simulink model "torqueWalking"  (Simulink 8.9)
settings: Solver=FixedStepDiscrete  StartTime=0.0  StopTime=Config.t_end  FixedStep=Config.t_step  RelTol=1e-3  EnableMultiTasking=on
InitFcn:
  | cd(fileparts(which(bdroot)));
  | initTorqueWalkingMPC;
undefined symbols (not defined in the file or in its folder): biasVectorConstraint_feet, Config, ConstraintMatrix_feet, DiscIntNeverNeededParam, Gains, ROBOT_DOF, Sat
libraries: WBToolboxLibrary x101
(part 1 of 3)
settings Model: SuppressorTable=22 serialization::archive 11 0 6 0 0 0 11 0  Creator=gnava  LastModifiedBy=mcharbonneau
settings DataIOCC: LimitDataPoints=off  SaveFormat=Dataset  SignalLoggingSaveFormat=Dataset
settings OptimizationCC: LifeSpan=auto
settings DebuggingCC: UnderspecifiedInitializationDetection=Simplified  MergeDetectMultiDrivingBlocksExec=error  FcnCallInpInsideContextMsg=error  StateNameClashWarn=none  SFUnexpectedBacktrackingDiag=error  SFNoUnconditionalDefaultTransitionDiag=error
settings HardwareCC: ProdBitPerPointer=64  ProdBitPerSizeT=64  ProdBitPerPtrDiffT=64  ProdLargestAtomicFloat=Float  ProdIntDivRoundTo=Zero  ProdEndianess=LittleEndian  ProdWordSize=64  ProdHWDeviceType=Intel->x86-64 (Windows64)
settings ModelReferenceCC: PropagateSignalLabelsOutOfModel=on
settings GRTTargetCC: TargetLangStandard=C99 (ISO)  GeneratePreprocessorConditionals=Use local settings  CombineOutputUpdateFcns=on  GRTInterface=off
settings ConfigComp: CovSFcnEnable=off

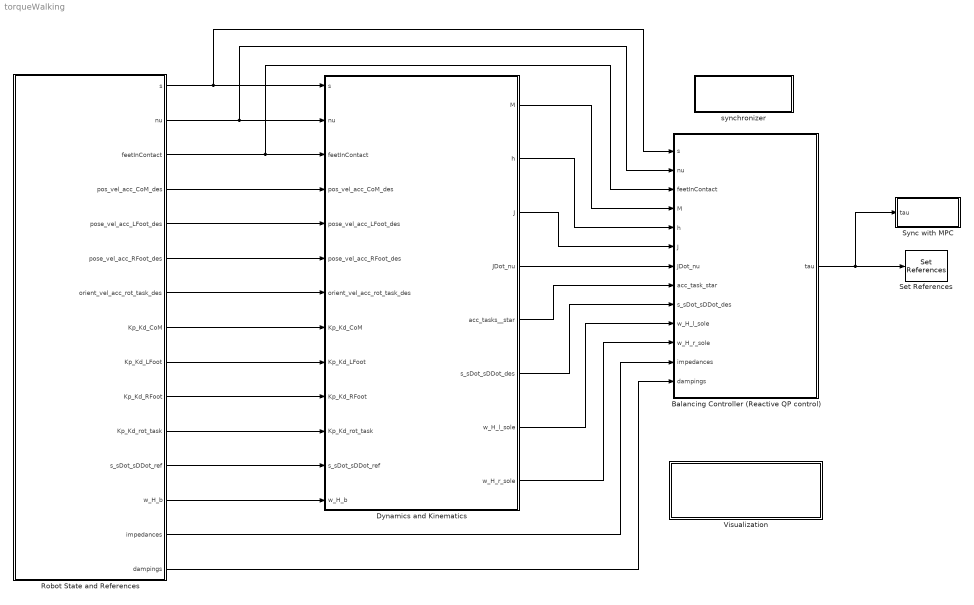
== system torqueWalking ==
  Balancing Controller (Reactive QP control) : Subsystem
  Dynamics and Kinematics : Subsystem
  Robot State and References : Subsystem
  Set References : WBToolboxLibrary/wholeBodyActuators/Set References  controlType=Torque  fullOrSubControl=Full  controlledJoints=''  robotName=WBT_robotName  localName=WBT_modelName  wbiFile=WBT_wbiFilename  wbiList=WBT_wbiList
      settings: SourceProductName=Whole Body Toolbox
  Sync with MPC : Subsystem
      mask Display: disp('Sync with MPC')
  Visualization : Subsystem
      mask Display: disp('VISUALIZE AND DUMP DATA')
  synchronizer : Subsystem
      mask Display: disp('SYNCHRONIZER')
  wires:
  Robot State and References/2(nu) -> Dynamics and Kinematics/2(nu), Balancing Controller (Reactive QP control)/2(nu)
  Robot State and References/3(feetInContact) -> Balancing Controller (Reactive QP control)/3(feetInContact), Dynamics and Kinematics/3(feetInContact)
  Robot State and References/4(pos_vel_acc_CoM_des) -> Dynamics and Kinematics/4(pos_vel_acc_CoM_des)
  Robot State and References/5(pose_vel_acc_LFoot_des) -> Dynamics and Kinematics/5(pose_vel_acc_LFoot_des)
  Robot State and References/6(pose_vel_acc_RFoot_des) -> Dynamics and Kinematics/6(pose_vel_acc_RFoot_des)
  Robot State and References/7(orient_vel_acc_rot_task_des) -> Dynamics and Kinematics/7(orient_vel_acc_rot_task_des)
  Robot State and References/8(Kp_Kd_CoM) -> Dynamics and Kinematics/8(Kp_Kd_CoM)
  Robot State and References/9(Kp_Kd_LFoot) -> Dynamics and Kinematics/9(Kp_Kd_LFoot)
  Robot State and References/10(Kp_Kd_RFoot) -> Dynamics and Kinematics/10(Kp_Kd_RFoot)
  Robot State and References/11(Kp_Kd_rot_task) -> Dynamics and Kinematics/11(Kp_Kd_rot_task)
  Robot State and References/12(s_sDot_sDDot_ref) -> Dynamics and Kinematics/12(s_sDot_sDDot_ref)
  Robot State and References/13(w_H_b) -> Dynamics and Kinematics/13(w_H_b)
  Dynamics and Kinematics/4(JDot_nu) -> Balancing Controller (Reactive QP control)/7(JDot_nu)
  Robot State and References/1(s) -> Dynamics and Kinematics/1(s), Balancing Controller (Reactive QP control)/1(s)
  Dynamics and Kinematics/1(M) -> Balancing Controller (Reactive QP control)/4(M)
  Dynamics and Kinematics/2(h) -> Balancing Controller (Reactive QP control)/5(h)
  Dynamics and Kinematics/3(J) -> Balancing Controller (Reactive QP control)/6(J)
  Balancing Controller (Reactive QP control)/1(tau) -> Sync with MPC/1(tau), Set References/1
  Dynamics and Kinematics/5(acc_tasks__star) -> Balancing Controller (Reactive QP control)/8(acc_task_star)
  Dynamics and Kinematics/6(s_sDot_sDDot_des) -> Balancing Controller (Reactive QP control)/9(s_sDot_sDDot_des)
  Dynamics and Kinematics/7(w_H_l_sole) -> Balancing Controller (Reactive QP control)/10(w_H_l_sole)
  Dynamics and Kinematics/8(w_H_r_sole) -> Balancing Controller (Reactive QP control)/11(w_H_r_sole)
  Robot State and References/14(impedances) -> Balancing Controller (Reactive QP control)/12(impedances)
  Robot State and References/15(dampings) -> Balancing Controller (Reactive QP control)/13(dampings)

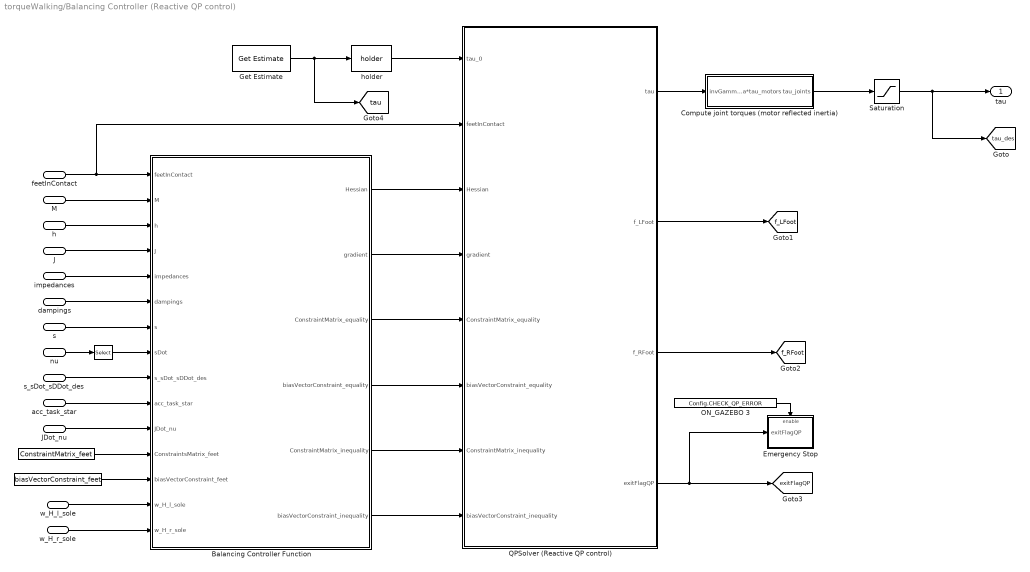
== system torqueWalking/Balancing Controller (Reactive QP control) ==
  s : Inport
  nu : Inport  Port=2
  feetInContact : Inport  Port=3
  M : Inport  Port=4
  h : Inport  Port=5
  J : Inport  Port=6
  JDot_nu : Inport  Port=7
  acc_task_star : Inport  Port=8
  s_sDot_sDDot_des : Inport  Port=9
  w_H_l_sole : Inport  Port=10
  w_H_r_sole : Inport  Port=11
  impedances : Inport  Port=12
  dampings : Inport  Port=13
  "   " : Constant  Value=ConstraintMatrix_feet
  "      " : Constant  Value=biasVectorConstraint_feet
  "             " : Selector  InputPortWidth=ROBOT_DOF+6  IndexOptions=Index vector (dialog)  Indices=[7:ROBOT_DOF+6]  OutputSizes=1
  Balancing Controller Function : MATLAB Function  TreatAsAtomicUnit=on
  Compute joint torques (motor reflected inertia) : Subsystem
  Emergency Stop : Subsystem
  Get Estimate : WBToolboxLibrary/wholeBodyStates/Get Estimate  estimateType=Joints Torque  robotName=WBT_robotName  localName=WBT_modelName  wbiFile=WBT_wbiFilename  wbiList=WBT_wbiList
      settings: SourceProductName=Whole Body Toolbox
  ON_GAZEBO 3 : Constant  Value=Config.CHECK_QP_ERROR
  QPSolver (Reactive QP control) : Subsystem
  Saturation : Saturate  UpperLimit=Sat.tau_max  LowerLimit=-Sat.tau_max
  "holder " : WBToolboxLibrary/Utilities/holder 
      settings: SourceProductName=Whole Body Toolbox
  tau : Outport
  tag scope: exitFlagQP=global, f_LFoot=global, f_RFoot=global, tau=global, tau_des=global
  wires:
  QPSolver (Reactive QP control)/1(tau) -> Compute joint torques (motor reflected inertia)/1(invGamma*tau_motors)
  "holder "/1 -> QPSolver (Reactive QP control)/1(tau_0)
  Balancing Controller Function/3(ConstraintMatrix_equality) -> QPSolver (Reactive QP control)/5(ConstraintMatrix_equality)
  Balancing Controller Function/6(biasVectorConstraint_inequality) -> QPSolver (Reactive QP control)/8(biasVectorConstraint_inequality)
  Balancing Controller Function/2(gradient) -> QPSolver (Reactive QP control)/4(gradient)
  Balancing Controller Function/4(biasVectorConstraint_equality) -> QPSolver (Reactive QP control)/6(biasVectorConstraint_equality)
  Balancing Controller Function/5(ConstraintMatrix_inequality) -> QPSolver (Reactive QP control)/7(ConstraintMatrix_inequality)
  w_H_r_sole/1 -> Balancing Controller Function/15(w_H_r_sole)
  w_H_l_sole/1 -> Balancing Controller Function/14(w_H_l_sole)
  "      "/1 -> Balancing Controller Function/13(biasVectorConstraint_feet)
  "   "/1 -> Balancing Controller Function/12(ConstraintsMatrix_feet)
  JDot_nu/1 -> Balancing Controller Function/11(JDot_nu)
  acc_task_star/1 -> Balancing Controller Function/10(acc_task_star)
  s_sDot_sDDot_des/1 -> Balancing Controller Function/9(s_sDot_sDDot_des)
  nu/1 -> "             "/1
  s/1 -> Balancing Controller Function/7(s)
  dampings/1 -> Balancing Controller Function/6(dampings)
  impedances/1 -> Balancing Controller Function/5(impedances)
  J/1 -> Balancing Controller Function/4(J)
  h/1 -> Balancing Controller Function/3(h)
  M/1 -> Balancing Controller Function/2(M)
  Get Estimate/1 -> [tau], "holder "/1
  "             "/1 -> Balancing Controller Function/8(sDot)
  Saturation/1 -> tau/1, [tau_des]
  Balancing Controller Function/1(Hessian) -> QPSolver (Reactive QP control)/3(Hessian)
  feetInContact/1 -> Balancing Controller Function/1(feetInContact), QPSolver (Reactive QP control)/2(feetInContact)
  QPSolver (Reactive QP control)/2(f_LFoot) -> [f_LFoot]
  QPSolver (Reactive QP control)/3(f_RFoot) -> [f_RFoot]
  QPSolver (Reactive QP control)/4(exitFlagQP) -> Emergency Stop/1(exitFlagQP), [exitFlagQP]
  ON_GAZEBO 3/1 -> Emergency Stop/Enable
  Compute joint torques (motor reflected inertia)/1(tau_joints) -> Saturation/1

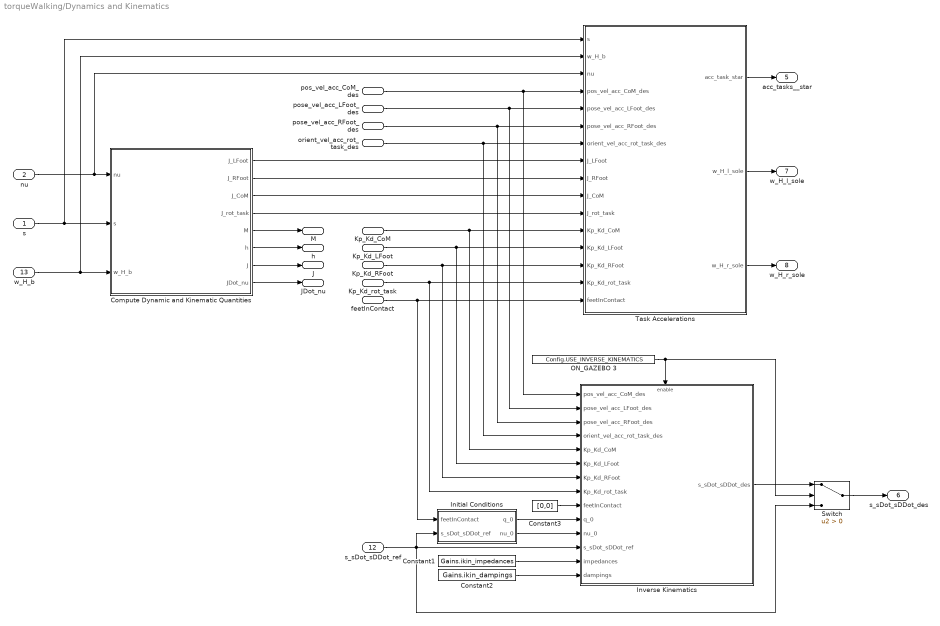
== system torqueWalking/Dynamics and Kinematics ==
  s : Inport
  nu : Inport  Port=2
  feetInContact : Inport  Port=3
  pos_vel_acc_CoM_des : Inport  Port=4
  pose_vel_acc_LFoot_des : Inport  Port=5
  pose_vel_acc_RFoot_des : Inport  Port=6
  orient_vel_acc_rot_task_des : Inport  Port=7
  Kp_Kd_CoM : Inport  Port=8
  Kp_Kd_LFoot : Inport  Port=9
  Kp_Kd_RFoot : Inport  Port=10
  Kp_Kd_rot_task : Inport  Port=11
  s_sDot_sDDot_ref : Inport  Port=12
  w_H_b : Inport  Port=13
  Compute Dynamic and Kinematic Quantities : Subsystem
  Constant1 : Constant  Value=Gains.ikin_impedances
  Constant2 : Constant  Value=Gains.ikin_dampings
  Constant3 : Constant  Value=[0,0]
  Initial Conditions : Subsystem
  Inverse Kinematics : Subsystem
  ON_GAZEBO 3 : Constant  Value=Config.USE_INVERSE_KINEMATICS
  Switch : Switch  Criteria=u2 > Threshold
  Task Accelerations : Subsystem
  M : Outport
  h : Outport  Port=2
  J : Outport  Port=3
  JDot_nu : Outport  Port=4
  acc_tasks__star : Outport  Port=5
  s_sDot_sDDot_des : Outport  Port=6
  w_H_l_sole : Outport  Port=7
  w_H_r_sole : Outport  Port=8
  wires:
  pos_vel_acc_CoM_des/1 -> Task Accelerations/4(pos_vel_acc_CoM_des), Inverse Kinematics/1(pos_vel_acc_CoM_des)
  pose_vel_acc_LFoot_des/1 -> Task Accelerations/5(pose_vel_acc_LFoot_des), Inverse Kinematics/2(pose_vel_acc_LFoot_des)
  pose_vel_acc_RFoot_des/1 -> Task Accelerations/6(pose_vel_acc_RFoot_des), Inverse Kinematics/3(pose_vel_acc_RFoot_des)
  orient_vel_acc_rot_task_des/1 -> Task Accelerations/7(orient_vel_acc_rot_task_des), Inverse Kinematics/4(orient_vel_acc_rot_task_des)
  Kp_Kd_CoM/1 -> Task Accelerations/12(Kp_Kd_CoM), Inverse Kinematics/5(Kp_Kd_CoM)
  Kp_Kd_LFoot/1 -> Task Accelerations/13(Kp_Kd_LFoot), Inverse Kinematics/6(Kp_Kd_LFoot)
  Kp_Kd_RFoot/1 -> Task Accelerations/14(Kp_Kd_RFoot), Inverse Kinematics/7(Kp_Kd_RFoot)
  Kp_Kd_rot_task/1 -> Task Accelerations/15(Kp_Kd_rot_task), Inverse Kinematics/8(Kp_Kd_rot_task)
  Task Accelerations/1(acc_task_star) -> acc_tasks__star/1
  ON_GAZEBO 3/1 -> Switch/2, Inverse Kinematics/Enable
  Inverse Kinematics/1(s_sDot_sDDot_des) -> Switch/1
  nu/1 -> Compute Dynamic and Kinematic Quantities/1(nu), Task Accelerations/3(nu)
  s/1 -> Task Accelerations/1(s), Compute Dynamic and Kinematic Quantities/2(s)
  w_H_b/1 -> Compute Dynamic and Kinematic Quantities/3(w_H_b), Task Accelerations/2(w_H_b)
  Compute Dynamic and Kinematic Quantities/6(h) -> h/1
  Compute Dynamic and Kinematic Quantities/1(J_LFoot) -> Task Accelerations/8(J_LFoot)
  Compute Dynamic and Kinematic Quantities/2(J_RFoot) -> Task Accelerations/9(J_RFoot)
  Compute Dynamic and Kinematic Quantities/3(J_CoM) -> Task Accelerations/10(J_CoM)
  Compute Dynamic and Kinematic Quantities/5(M) -> M/1
  Compute Dynamic and Kinematic Quantities/4(J_rot_task) -> Task Accelerations/11(J_rot_task)
  Compute Dynamic and Kinematic Quantities/7(J) -> J/1
  Compute Dynamic and Kinematic Quantities/8(JDot_nu) -> JDot_nu/1
  s_sDot_sDDot_ref/1 -> Switch/3, Inverse Kinematics/12(s_sDot_sDDot_ref), Initial Conditions/2(s_sDot_sDDot_ref)
  Initial Conditions/1(q_0) -> Inverse Kinematics/10(q_0)
  Initial Conditions/2(nu_0) -> Inverse Kinematics/11(nu_0)
  Constant1/1 -> Inverse Kinematics/13(impedances)
  Constant2/1 -> Inverse Kinematics/14(dampings)
  Switch/1 -> s_sDot_sDDot_des/1
  Constant3/1 -> Inverse Kinematics/9(feetInContact)
  feetInContact/1 -> Initial Conditions/1(feetInContact), Task Accelerations/16(feetInContact)
  Task Accelerations/2(w_H_l_sole) -> w_H_l_sole/1
  Task Accelerations/3(w_H_r_sole) -> w_H_r_sole/1

== system torqueWalking/Robot State and References ==
  Gain Scheduling : Subsystem
  "Smooth References " : Subsystem
  State Machines : Subsystem
  s : Outport
  nu : Outport  Port=2
  feetInContact : Outport  Port=3
  pos_vel_acc_CoM_des : Outport  Port=4
  pose_vel_acc_LFoot_des : Outport  Port=5
  pose_vel_acc_RFoot_des : Outport  Port=6
  orient_vel_acc_rot_task_des : Outport  Port=7
  Kp_Kd_CoM : Outport  Port=8
  Kp_Kd_LFoot : Outport  Port=9
  Kp_Kd_RFoot : Outport  Port=10
  Kp_Kd_rot_task : Outport  Port=11
  s_sDot_sDDot_ref : Outport  Port=12
  w_H_b : Outport  Port=13
  impedances : Outport  Port=14
  dampings : Outport  Port=15
  wires:
  Gain Scheduling/1(Kp_Kd_CoM) -> Kp_Kd_CoM/1
  Gain Scheduling/2(Kp_Kd_LFoot) -> Kp_Kd_LFoot/1
  Gain Scheduling/3(Kp_Kd_RFoot) -> Kp_Kd_RFoot/1
  Gain Scheduling/4(Kp_Kd_rot_task) -> Kp_Kd_rot_task/1
  Gain Scheduling/5(impedances) -> impedances/1
  Gain Scheduling/6(dampings) -> dampings/1
  State Machines/5(state) -> Gain Scheduling/1(state), "Smooth References "/1(state)
  State Machines/4(feetInContact) -> feetInContact/1
  State Machines/3(nu) -> nu/1
  State Machines/2(w_H_b) -> w_H_b/1
  State Machines/6(references_CoM) -> "Smooth References "/2(references_CoM)
  State Machines/7(references_LFoot) -> "Smooth References "/3(references_LFoot)
  State Machines/8(references_RFoot) -> "Smooth References "/4(references_RFoot)
  State Machines/9(references_rot_task) -> "Smooth References "/5(references_rot_task)
  State Machines/10(references_s) -> "Smooth References "/6(references_s)
  "Smooth References "/1(pos_vel_acc_CoM_des) -> pos_vel_acc_CoM_des/1
  "Smooth References "/2(pose_vel_acc_LFoot_des) -> pose_vel_acc_LFoot_des/1
  "Smooth References "/3(pose_vel_acc_RFoot_des) -> pose_vel_acc_RFoot_des/1
  "Smooth References "/4(orient_vel_acc_rot_task_des) -> orient_vel_acc_rot_task_des/1
  "Smooth References "/5(s_sDot_sDDot_ref) -> s_sDot_sDDot_ref/1
  State Machines/1(s) -> s/1

== system torqueWalking/Sync with MPC ==
  tau : Inport
  Clock : Clock
  Gain : Gain  Gain=0
  Mux : Mux  Inputs=2
  Selector : Selector  InputPortWidth=ROBOT_DOF  IndexOptions=Index vector (dialog)  Indices=[1]  OutputSizes=1
  Yarp Write : WBToolboxLibrary/Utilities/Yarp Write  portName=PORTS.ACK  autoconnect=on  errorOnConnection=off
      settings: SourceProductName=Whole Body Toolbox
  wires:
  Clock/1 -> Mux/2
  tau/1 -> Selector/1
  Mux/1 -> Yarp Write/1
  Selector/1 -> Gain/1
  Gain/1 -> Mux/1

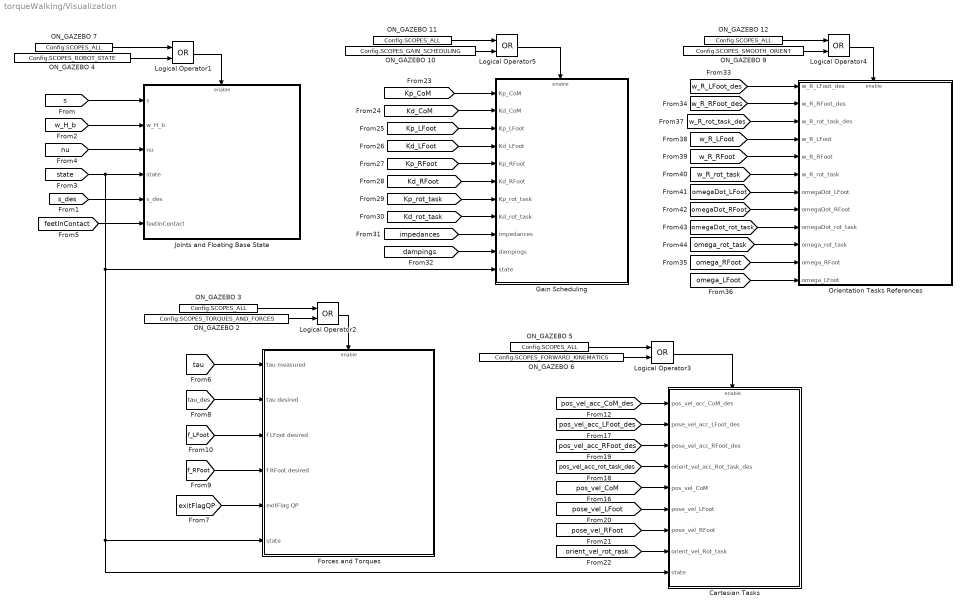
== system torqueWalking/Visualization ==
  Cartesian Tasks : Subsystem
  Forces and Torques : Subsystem
  Gain Scheduling : Subsystem
  Joints and Floating Base State : Subsystem
  Logical Operator{1..5} (5 alike) : Logic  Operator=OR  AllPortsSameDT=off  OutDataTypeStr=boolean
  ON_GAZEBO 10 : Constant  Value=Config.SCOPES_GAIN_SCHEDULING
  ON_GAZEBO {3,5,7,11..12} (5 alike) : Constant  Value=Config.SCOPES_ALL
  ON_GAZEBO 2 : Constant  Value=Config.SCOPES_TORQUES_AND_FORCES
  ON_GAZEBO 4 : Constant  Value=Config.SCOPES_ROBOT_STATE
  ON_GAZEBO 6 : Constant  Value=Config.SCOPES_FORWARD_KINEMATICS
  ON_GAZEBO 9 : Constant  Value=Config.SCOPES_SMOOTH_ORIENT
  Orientation Tasks References : Subsystem
  wires:
  [s] -> Joints and Floating Base State/1(s)
  [w_H_b] -> Joints and Floating Base State/2(w_H_b)
  [s_des] -> Joints and Floating Base State/5(s_des)
  [nu] -> Joints and Floating Base State/3(nu)
  [state] -> Cartesian Tasks/9(state), Forces and Torques/6(state), Gain Scheduling/11(state), Joints and Floating Base State/4(state)
  [tau] -> Forces and Torques/1(tau measured)
  [tau_des] -> Forces and Torques/2(tau desired)
  [f_LFoot] -> Forces and Torques/3(f LFoot desired)
  [f_RFoot] -> Forces and Torques/4(f RFoot desired)
  [exitFlagQP] -> Forces and Torques/5(exitFlag QP)
  ON_GAZEBO 4/1 -> Logical Operator1/2
  ON_GAZEBO 7/1 -> Logical Operator1/1
  Logical Operator1/1 -> Joints and Floating Base State/Enable
  [feetInContact] -> Joints and Floating Base State/6(feetInContact)
  Logical Operator2/1 -> Forces and Torques/Enable
  ON_GAZEBO 3/1 -> Logical Operator2/1
  ON_GAZEBO 2/1 -> Logical Operator2/2
  ON_GAZEBO 6/1 -> Logical Operator3/2
  Logical Operator3/1 -> Cartesian Tasks/Enable
  ON_GAZEBO 5/1 -> Logical Operator3/1
  [pos_vel_acc_CoM_des] -> Cartesian Tasks/1(pos_vel_acc_CoM_des)
  [pos_vel_acc_LFoot_des] -> Cartesian Tasks/2(pose_vel_acc_LFoot_des)
  [pos_vel_acc_RFoot_des] -> Cartesian Tasks/3(pose_vel_acc_RFoot_des)
  [pos_vel_acc_rot_task_des] -> Cartesian Tasks/4(orient_vel_acc_Rot_task_des)
  [pos_vel_CoM] -> Cartesian Tasks/5(pos_vel_CoM)
  [pose_vel_LFoot] -> Cartesian Tasks/6(pose_vel_LFoot)
  [pose_vel_RFoot] -> Cartesian Tasks/7(pose_vel_RFoot)
  [orient_vel_rot_rask] -> Cartesian Tasks/8(orient_vel_Rot_task)
  ON_GAZEBO 10/1 -> Logical Operator5/2
  ON_GAZEBO 11/1 -> Logical Operator5/1
  Logical Operator5/1 -> Gain Scheduling/Enable
  [Kp_CoM] -> Gain Scheduling/1(Kp_CoM)
  [Kd_CoM] -> Gain Scheduling/2(Kd_CoM)
  [Kp_LFoot] -> Gain Scheduling/3(Kp_LFoot)
  [Kd_LFoot] -> Gain Scheduling/4(Kd_LFoot)
  [Kp_RFoot] -> Gain Scheduling/5(Kp_RFoot)
  [Kd_RFoot] -> Gain Scheduling/6(Kd_RFoot)
  [Kp_rot_task] -> Gain Scheduling/7(Kp_rot_task)
  [Kd_rot_task] -> Gain Scheduling/8(Kd_rot_task)
  [impedances] -> Gain Scheduling/9(impedances)
  [dampings] -> Gain Scheduling/10(dampings)
  ON_GAZEBO 9/1 -> Logical Operator4/2
  ON_GAZEBO 12/1 -> Logical Operator4/1
  Logical Operator4/1 -> Orientation Tasks References/Enable
  [omega_LFoot] -> Orientation Tasks References/12(omega_LFoot)
  [omega_RFoot] -> Orientation Tasks References/11(omega_RFoot)
  [omega_rot_task] -> Orientation Tasks References/10(omega_rot_task)
  [omegaDot_RFoot] -> Orientation Tasks References/8(omegaDot_RFoot)
  [omegaDot_rot_task] -> Orientation Tasks References/9(omegaDot_rot_task)
  [omegaDot_LFoot] -> Orientation Tasks References/7(omegaDot_LFoot)
  [w_R_LFoot_des] -> Orientation Tasks References/1(w_R_LFoot_des)
  [w_R_RFoot_des] -> Orientation Tasks References/2(w_R_RFoot_des)
  [w_R_rot_task_des] -> Orientation Tasks References/3(w_R_rot_task_des)
  [w_R_LFoot] -> Orientation Tasks References/4(w_R_LFoot)
  [w_R_RFoot] -> Orientation Tasks References/5(w_R_RFoot)
  [w_R_rot_task] -> Orientation Tasks References/6(w_R_rot_task)

== system torqueWalking/synchronizer ==
  GAZEBO_SYNCHRONIZER : Subsystem
  Logical Operator : Logic  Operator=NOT  AllPortsSameDT=off  OutDataTypeStr=boolean
  "ON_GAZEBO " : Constant  Value=Config.ON_GAZEBO
  REAL_TIME_SYNC : Subsystem
  wires:
  Logical Operator/1 -> REAL_TIME_SYNC/Enable
  "ON_GAZEBO "/1 -> Logical Operator/1, GAZEBO_SYNCHRONIZER/Enable

== system torqueWalking/Balancing Controller (Reactive QP control)/Compute joint torques (motor reflected inertia) ==
  invGamma*tau_motors : Inport
  " " : Constant  Value=Config.USE_MOTOR_REFLECTED_INERTIA
  Add : Sum  Inputs=-+
  Gain : Gain  Gain=Config.K_ff
  Get Estimate : WBToolboxLibrary/wholeBodyStates/Get Estimate  estimateType=Joints Acceleration  robotName=WBT_robotName  localName=WBT_modelName  wbiFile=WBT_wbiFilename  wbiList=WBT_wbiList
      settings: SourceProductName=Whole Body Toolbox
  Motors Inertia : Constant  Value=Config.I_m
  Product : Product  Multiplication=Matrix(*)
  Product1 : Product  Multiplication=Matrix(*)
  Switch : Switch  Criteria=u2 > Threshold
  Transmission ratio : Constant  Value=Config.invGamma
  tau_joints : Outport
  wires:
  Product1/1 -> Product/1
  Get Estimate/1 -> Product/2
  Product/1 -> Gain/1
  Transmission ratio/1 -> Product1/1
  Motors Inertia/1 -> Product1/2
  Gain/1 -> Add/1
  Add/1 -> Switch/1
  " "/1 -> Switch/2
  Switch/1 -> tau_joints/1
  invGamma*tau_motors/1 -> Switch/3, Add/2

== system torqueWalking/Balancing Controller (Reactive QP control)/Emergency Stop ==
  exitFlagQP : Inport
  Enable : EnablePort
  Constant : Constant  Value=2
  Constant1 : Constant  Value=0  OutDataTypeStr=boolean
  Constant2 : Constant  OutDataTypeStr=boolean
  Stop Simulation : Stop
  Sum : Sum  Inputs=|++
  Switch : Switch  Criteria=u2 > Threshold  Threshold=0.1
  wires:
  exitFlagQP/1 -> Sum/1
  Sum/1 -> Switch/2
  Switch/1 -> Stop Simulation/1
  Constant/1 -> Sum/2
  Constant1/1 -> Switch/1
  Constant2/1 -> Switch/3

== system torqueWalking/Balancing Controller (Reactive QP control)/QPSolver (Reactive QP control) ==
  tau_0 : Inport
  feetInContact : Inport  Port=2
  Hessian : Inport  Port=3
  gradient : Inport  Port=4
  ConstraintMatrix_equality : Inport  Port=5
  biasVectorConstraint_equality : Inport  Port=6
  ConstraintMatrix_inequality : Inport  Port=7
  biasVectorConstraint_inequality : Inport  Port=8
  QPSolver : M-S-Function  FunctionName=QPBalancingMPC  Parameters=ROBOT_DOF, Sat, Config
  tau : Outport
  f_LFoot : Outport  Port=2
  f_RFoot : Outport  Port=3
  exitFlagQP : Outport  Port=4
  wires:
  gradient/1 -> QPSolver/4
  Hessian/1 -> QPSolver/3
  biasVectorConstraint_inequality/1 -> QPSolver/8
  feetInContact/1 -> QPSolver/2
  QPSolver/2 -> f_LFoot/1
  ConstraintMatrix_inequality/1 -> QPSolver/7
  biasVectorConstraint_equality/1 -> QPSolver/6
  ConstraintMatrix_equality/1 -> QPSolver/5
  tau_0/1 -> QPSolver/1
  QPSolver/1 -> tau/1
  QPSolver/3 -> f_RFoot/1
  QPSolver/4 -> exitFlagQP/1

== system torqueWalking/Dynamics and Kinematics/Compute Dynamic and Kinematic Quantities ==
  nu : Inport
  s : Inport  Port=2
  w_H_b : Inport  Port=3
  "  " : Selector  NumberOfDimensions=2  InputPortWidth=ROBOT_DOF+16  IndexOptions=Index vector (dialog),Index vector (dialog)  Indices=[1:3],[1:ROBOT_DOF+6]  OutputSizes=1,1
  "   " : Selector  InputPortWidth=6  IndexOptions=Index vector (dialog)  Indices=[1:3]  OutputSizes=1
  "     " : Selector  NumberOfDimensions=2  InputPortWidth=ROBOT_DOF+16  IndexOptions=Index vector (dialog),Index vector (dialog)  Indices=[4:6],[1:ROBOT_DOF+6]  OutputSizes=1,1
  "               " : Selector  InputPortWidth=6  IndexOptions=Index vector (dialog)  Indices=[4:6]  OutputSizes=1
  Jacobians and JDot_nu : Subsystem
  Mass Matrix and Bias Forces : Subsystem
  Matrix Concatenate : Concatenate  NumInputs=4  Mode=Multidimensional array
  Selector : Selector  InputPortWidth=ROBOT_DOF+6  IndexOptions=Index vector (dialog)  Indices=[1:6]  OutputSizes=1
  Selector1 : Selector  InputPortWidth=ROBOT_DOF+6  IndexOptions=Index vector (dialog)  Indices=[7:ROBOT_DOF+6]  OutputSizes=1
  Vector Concatenate : Concatenate  NumInputs=4
  J_LFoot : Outport
  J_RFoot : Outport  Port=2
  J_CoM : Outport  Port=3
  J_rot_task : Outport  Port=4
  M : Outport  Port=5
  h : Outport  Port=6
  J : Outport  Port=7
  JDot_nu : Outport  Port=8
  wires:
  "               "/1 -> Vector Concatenate/4
  "  "/1 -> J_CoM/1, Matrix Concatenate/3
  "     "/1 -> J_rot_task/1, Matrix Concatenate/4
  Vector Concatenate/1 -> JDot_nu/1
  Selector1/1 -> Mass Matrix and Bias Forces/3(sDot), Jacobians and JDot_nu/3(sDot)
  Matrix Concatenate/1 -> J/1
  nu/1 -> Selector/1, Selector1/1
  Selector/1 -> Mass Matrix and Bias Forces/2(nu_b), Jacobians and JDot_nu/2(nu_b)
  "   "/1 -> Vector Concatenate/3
  Mass Matrix and Bias Forces/2(M(q)) -> M/1
  Mass Matrix and Bias Forces/1(h(q,nu)) -> h/1
  s/1 -> Jacobians and JDot_nu/1(s), Mass Matrix and Bias Forces/1(s)
  w_H_b/1 -> Jacobians and JDot_nu/4(w_H_b), Mass Matrix and Bias Forces/4(w_H_b)
  Jacobians and JDot_nu/2(J_RFoot) -> J_RFoot/1, Matrix Concatenate/2
  Jacobians and JDot_nu/1(J_LFoot) -> J_LFoot/1, Matrix Concatenate/1
  Jacobians and JDot_nu/3(J_CoM) -> "  "/1
  Jacobians and JDot_nu/4(J_rot_task) -> "     "/1
  Jacobians and JDot_nu/5(JDot_nu_LFoot) -> Vector Concatenate/1
  Jacobians and JDot_nu/6(JDot_nu_RFoot) -> Vector Concatenate/2
  Jacobians and JDot_nu/7(JDot_nu_CoM) -> "   "/1
  Jacobians and JDot_nu/8(JDot_nu_rot_task) -> "               "/1

== system torqueWalking/Dynamics and Kinematics/Initial Conditions ==
  feetInContact : Inport
  s_sDot_sDDot_ref : Inport  Port=2
  "   1" : WBToolboxLibrary/Utilities/holder 
      settings: SourceProductName=Whole Body Toolbox
  "   2" : WBToolboxLibrary/Utilities/holder 
      settings: SourceProductName=Whole Body Toolbox
  Compute world to base transform : Subsystem
  Mux : Mux  Inputs=2
  Reshape : Reshape
  Selector : Selector  NumberOfDimensions=2  InputPortWidth=3  IndexOptions=Index vector (dialog),Index vector (dialog)  Indices=[1:ROBOT_DOF],1  OutputSizes=1,1
  Selector1 : Selector  NumberOfDimensions=2  InputPortWidth=3  IndexOptions=Index vector (dialog),Index vector (dialog)  Indices=[1:ROBOT_DOF],2  OutputSizes=1,1
  compute state velocity : Subsystem
  q_0 : Outport
  nu_0 : Outport  Port=2
  wires:
  Reshape/1 -> Mux/1
  Mux/1 -> q_0/1
  s_sDot_sDDot_ref/1 -> "   2"/1
  "   2"/1 -> Selector/1, Selector1/1
  Selector/1 -> Mux/2, compute state velocity/1(s), Compute world to base transform/1(s)
  compute state velocity/1(nu) -> nu_0/1
  feetInContact/1 -> "   1"/1
  Compute world to base transform/1(w_H_b) -> Reshape/1, compute state velocity/2(w_H_b)
  "   1"/1 -> compute state velocity/3("feetInContact ")
  Selector1/1 -> compute state velocity/4(sDot)

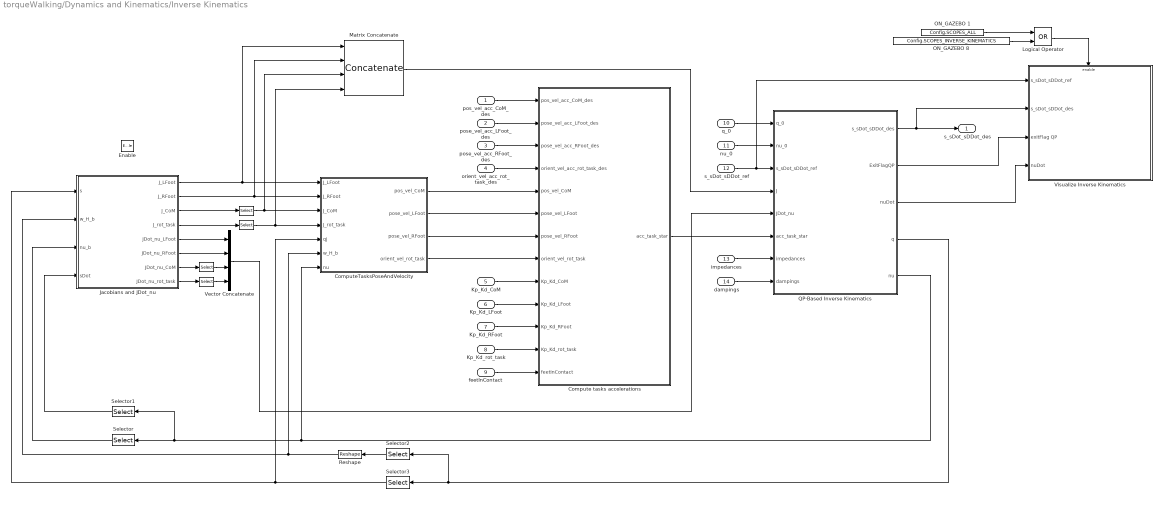
== system torqueWalking/Dynamics and Kinematics/Inverse Kinematics ==
  pos_vel_acc_CoM_des : Inport
  pose_vel_acc_LFoot_des : Inport  Port=2
  pose_vel_acc_RFoot_des : Inport  Port=3
  orient_vel_acc_rot_task_des : Inport  Port=4
  Kp_Kd_CoM : Inport  Port=5
  Kp_Kd_LFoot : Inport  Port=6
  Kp_Kd_RFoot : Inport  Port=7
  Kp_Kd_rot_task : Inport  Port=8
  feetInContact : Inport  Port=9
  q_0 : Inport  Port=10
  nu_0 : Inport  Port=11
  s_sDot_sDDot_ref : Inport  Port=12
  impedances : Inport  Port=13
  dampings : Inport  Port=14
  Enable : EnablePort
  "  " : Selector  NumberOfDimensions=2  InputPortWidth=ROBOT_DOF+16  IndexOptions=Index vector (dialog),Index vector (dialog)  Indices=[1:3],[1:ROBOT_DOF+6]  OutputSizes=1,1
  "   " : Selector  InputPortWidth=6  IndexOptions=Index vector (dialog)  Indices=[1:3]  OutputSizes=1
  "     " : Selector  NumberOfDimensions=2  InputPortWidth=ROBOT_DOF+16  IndexOptions=Index vector (dialog),Index vector (dialog)  Indices=[4:6],[1:ROBOT_DOF+6]  OutputSizes=1,1
  "               " : Selector  InputPortWidth=6  IndexOptions=Index vector (dialog)  Indices=[4:6]  OutputSizes=1
  Compute tasks accelerations : MATLAB Function  TreatAsAtomicUnit=on
  ComputeTasksPoseAndVelocity : Subsystem
  Jacobians and JDot_nu : Subsystem
  Logical Operator : Logic  Operator=OR  AllPortsSameDT=off  OutDataTypeStr=boolean
  Matrix Concatenate : Concatenate  NumInputs=4  Mode=Multidimensional array
  ON_GAZEBO 1 : Constant  Value=Config.SCOPES_ALL
  ON_GAZEBO 8 : Constant  Value=Config.SCOPES_INVERSE_KINEMATICS
  QP-Based Inverse Kinematics : Subsystem
  Reshape : Reshape  OutputDimensionality=Customize  OutputDimensions=[4,4]
  Selector : Selector  InputPortWidth=ROBOT_DOF+6  IndexOptions=Index vector (dialog)  Indices=[1:6]  OutputSizes=1
  Selector1 : Selector  InputPortWidth=ROBOT_DOF+6  IndexOptions=Index vector (dialog)  Indices=[7:ROBOT_DOF+6]  OutputSizes=1
  Selector2 : Selector  InputPortWidth=ROBOT_DOF+16  IndexOptions=Index vector (dialog)  Indices=[1:16]  OutputSizes=1
  Selector3 : Selector  InputPortWidth=ROBOT_DOF+16  IndexOptions=Index vector (dialog)  Indices=[17:ROBOT_DOF+16]  OutputSizes=1
  Vector Concatenate : Concatenate  NumInputs=4
  Visualize Inverse Kinematics : Subsystem
  s_sDot_sDDot_des : Outport
  wires:
  Kp_Kd_CoM/1 -> Compute tasks accelerations/9(Kp_Kd_CoM)
  Kp_Kd_LFoot/1 -> Compute tasks accelerations/10(Kp_Kd_LFoot)
  pose_vel_acc_LFoot_des/1 -> Compute tasks accelerations/2(pose_vel_acc_LFoot_des)
  Kp_Kd_RFoot/1 -> Compute tasks accelerations/11(Kp_Kd_RFoot)
  orient_vel_acc_rot_task_des/1 -> Compute tasks accelerations/4(orient_vel_acc_rot_task_des)
  pose_vel_acc_RFoot_des/1 -> Compute tasks accelerations/3(pose_vel_acc_RFoot_des)
  Kp_Kd_rot_task/1 -> Compute tasks accelerations/12(Kp_Kd_rot_task)
  pos_vel_acc_CoM_des/1 -> Compute tasks accelerations/1(pos_vel_acc_CoM_des)
  ComputeTasksPoseAndVelocity/1(pos_vel_CoM) -> Compute tasks accelerations/5(pos_vel_CoM)
  ComputeTasksPoseAndVelocity/2(pose_vel_LFoot) -> Compute tasks accelerations/6(pose_vel_LFoot)
  ComputeTasksPoseAndVelocity/3(pose_vel_RFoot) -> Compute tasks accelerations/7(pose_vel_RFoot)
  ComputeTasksPoseAndVelocity/4(orient_vel_rot_task) -> Compute tasks accelerations/8(orient_vel_rot_task)
  s_sDot_sDDot_ref/1 -> Visualize Inverse Kinematics/1(s_sDot_sDDot_ref), QP-Based Inverse Kinematics/3(s_sDot_sDDot_ref)
  Selector2/1 -> Reshape/1
  "  "/1 -> ComputeTasksPoseAndVelocity/3(J_CoM), Matrix Concatenate/3
  "   "/1 -> Vector Concatenate/3
  Jacobians and JDot_nu/2(J_RFoot) -> Matrix Concatenate/2, ComputeTasksPoseAndVelocity/2(J_RFoot)
  Jacobians and JDot_nu/1(J_LFoot) -> Matrix Concatenate/1, ComputeTasksPoseAndVelocity/1(J_LFoot)
  Selector1/1 -> Jacobians and JDot_nu/4(sDot)
  Selector/1 -> Jacobians and JDot_nu/3(nu_b)
  Jacobians and JDot_nu/4(J_rot_task) -> "     "/1
  Jacobians and JDot_nu/5(JDot_nu_LFoot) -> Vector Concatenate/1
  Jacobians and JDot_nu/6(JDot_nu_RFoot) -> Vector Concatenate/2
  Jacobians and JDot_nu/7(JDot_nu_CoM) -> "   "/1
  Jacobians and JDot_nu/8(JDot_nu_rot_task) -> "               "/1
  Vector Concatenate/1 -> QP-Based Inverse Kinematics/5(JDot_nu)
  dampings/1 -> QP-Based Inverse Kinematics/8(dampings)
  Compute tasks accelerations/1(acc_task_star) -> QP-Based Inverse Kinematics/6(acc_task_star)
  impedances/1 -> QP-Based Inverse Kinematics/7(impedances)
  Matrix Concatenate/1 -> QP-Based Inverse Kinematics/4(J)
  nu_0/1 -> QP-Based Inverse Kinematics/2(nu_0)
  q_0/1 -> QP-Based Inverse Kinematics/1(q_0)
  QP-Based Inverse Kinematics/5(nu) -> ComputeTasksPoseAndVelocity/7(nu), Selector1/1, Selector/1
  QP-Based Inverse Kinematics/4(q) -> Selector2/1, Selector3/1
  QP-Based Inverse Kinematics/1(s_sDot_sDDot_des) -> Visualize Inverse Kinematics/2(s_sDot_sDDot_des), s_sDot_sDDot_des/1
  "     "/1 -> Matrix Concatenate/4, ComputeTasksPoseAndVelocity/4(J_rot_task)
  "               "/1 -> Vector Concatenate/4
  Jacobians and JDot_nu/3(J_CoM) -> "  "/1
  Reshape/1 -> Jacobians and JDot_nu/2(w_H_b), ComputeTasksPoseAndVelocity/6(w_H_b)
  Selector3/1 -> Jacobians and JDot_nu/1(s), ComputeTasksPoseAndVelocity/5(qj)
  feetInContact/1 -> Compute tasks accelerations/13(feetInContact)
  ON_GAZEBO 8/1 -> Logical Operator/2
  ON_GAZEBO 1/1 -> Logical Operator/1
  Logical Operator/1 -> Visualize Inverse Kinematics/Enable
  QP-Based Inverse Kinematics/2(ExitFlagQP) -> Visualize Inverse Kinematics/3(exitFlag QP)
  QP-Based Inverse Kinematics/3(nuDot) -> Visualize Inverse Kinematics/4(nuDot)

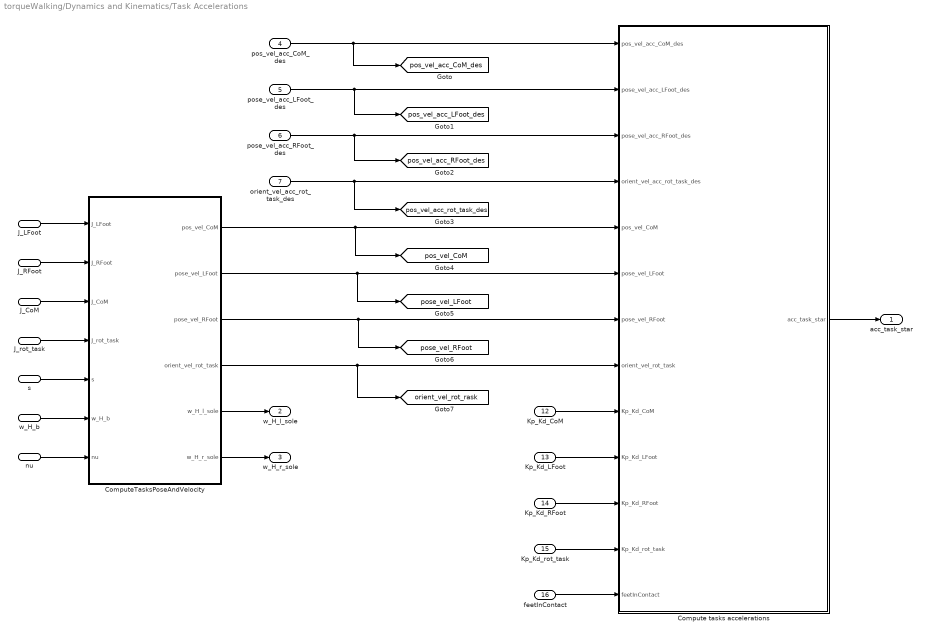
== system torqueWalking/Dynamics and Kinematics/Task Accelerations ==
  s : Inport
  w_H_b : Inport  Port=2
  nu : Inport  Port=3
  pos_vel_acc_CoM_des : Inport  Port=4
  pose_vel_acc_LFoot_des : Inport  Port=5
  pose_vel_acc_RFoot_des : Inport  Port=6
  orient_vel_acc_rot_task_des : Inport  Port=7
  J_LFoot : Inport  Port=8
  J_RFoot : Inport  Port=9
  J_CoM : Inport  Port=10
  J_rot_task : Inport  Port=11
  Kp_Kd_CoM : Inport  Port=12
  Kp_Kd_LFoot : Inport  Port=13
  Kp_Kd_RFoot : Inport  Port=14
  Kp_Kd_rot_task : Inport  Port=15
  feetInContact : Inport  Port=16
  Compute tasks accelerations : MATLAB Function  TreatAsAtomicUnit=on
  ComputeTasksPoseAndVelocity : Subsystem
  acc_task_star : Outport
  w_H_l_sole : Outport  Port=2
  w_H_r_sole : Outport  Port=3
  tag scope: orient_vel_rot_rask=global, pos_vel_CoM=global, pos_vel_acc_CoM_des=global, pos_vel_acc_LFoot_des=global, pos_vel_acc_RFoot_des=global, pos_vel_acc_rot_task_des=global, pose_vel_LFoot=global, pose_vel_RFoot=global
  wires:
  pos_vel_acc_CoM_des/1 -> [pos_vel_acc_CoM_des], Compute tasks accelerations/1(pos_vel_acc_CoM_des)
  Kp_Kd_RFoot/1 -> Compute tasks accelerations/11(Kp_Kd_RFoot)
  Kp_Kd_rot_task/1 -> Compute tasks accelerations/12(Kp_Kd_rot_task)
  feetInContact/1 -> Compute tasks accelerations/13(feetInContact)
  pose_vel_acc_RFoot_des/1 -> [pos_vel_acc_RFoot_des], Compute tasks accelerations/3(pose_vel_acc_RFoot_des)
  Kp_Kd_LFoot/1 -> Compute tasks accelerations/10(Kp_Kd_LFoot)
  Kp_Kd_CoM/1 -> Compute tasks accelerations/9(Kp_Kd_CoM)
  orient_vel_acc_rot_task_des/1 -> [pos_vel_acc_rot_task_des], Compute tasks accelerations/4(orient_vel_acc_rot_task_des)
  pose_vel_acc_LFoot_des/1 -> [pos_vel_acc_LFoot_des], Compute tasks accelerations/2(pose_vel_acc_LFoot_des)
  Compute tasks accelerations/1(acc_task_star) -> acc_task_star/1
  ComputeTasksPoseAndVelocity/1(pos_vel_CoM) -> [pos_vel_CoM], Compute tasks accelerations/5(pos_vel_CoM)
  ComputeTasksPoseAndVelocity/4(orient_vel_rot_task) -> [orient_vel_rot_rask], Compute tasks accelerations/8(orient_vel_rot_task)
  J_LFoot/1 -> ComputeTasksPoseAndVelocity/1(J_LFoot)
  J_RFoot/1 -> ComputeTasksPoseAndVelocity/2(J_RFoot)
  J_CoM/1 -> ComputeTasksPoseAndVelocity/3(J_CoM)
  J_rot_task/1 -> ComputeTasksPoseAndVelocity/4(J_rot_task)
  s/1 -> ComputeTasksPoseAndVelocity/5(s)
  w_H_b/1 -> ComputeTasksPoseAndVelocity/6(w_H_b)
  nu/1 -> ComputeTasksPoseAndVelocity/7(nu)
  ComputeTasksPoseAndVelocity/2(pose_vel_LFoot) -> [pose_vel_LFoot], Compute tasks accelerations/6(pose_vel_LFoot)
  ComputeTasksPoseAndVelocity/3(pose_vel_RFoot) -> [pose_vel_RFoot], Compute tasks accelerations/7(pose_vel_RFoot)
  ComputeTasksPoseAndVelocity/5(w_H_l_sole) -> w_H_l_sole/1
  ComputeTasksPoseAndVelocity/6(w_H_r_sole) -> w_H_r_sole/1

== system torqueWalking/Robot State and References/Gain Scheduling ==
  state : Inport
  Demux : Demux  Outputs=[6;12;12;6;ROBOT_DOF;ROBOT_DOF]
  Gain Scheduling Function : MATLAB Function  TreatAsAtomicUnit=on
  Minimum Jerk Trajectory Generator5 : WBToolboxLibrary/Utilities/Minimum Jerk Trajectory Generator  externalSettlingTime=on  settlingTime=3  sampleTime=Config.t_step  resetOnSettlingTime=off  firstDerivatives=off  secondDerivatives=off  explicitInitialValue=off
      settings: SourceProductName=Whole Body Toolbox
  Mux : Mux  Inputs=10
  Reshape : Reshape  OutputDimensionality=Customize  OutputDimensions=[3;2]
  Reshape1 : Reshape  OutputDimensionality=Customize  OutputDimensions=[6;2]
  Reshape2 : Reshape  OutputDimensionality=Customize  OutputDimensions=[6;2]
  Reshape3 : Reshape  OutputDimensionality=Customize  OutputDimensions=[3;2]
  Kp_Kd_CoM : Outport
  Kp_Kd_LFoot : Outport  Port=2
  Kp_Kd_RFoot : Outport  Port=3
  Kp_Kd_rot_task : Outport  Port=4
  impedances : Outport  Port=5
  dampings : Outport  Port=6
  tag scope: Kd_CoM=global, Kd_LFoot=global, Kd_RFoot=global, Kd_rot_task=global, Kp_CoM=global, Kp_LFoot=global, Kp_RFoot=global, Kp_rot_task=global, dampings=global, impedances=global
  wires:
  state/1 -> Gain Scheduling Function/1(state)
  Gain Scheduling Function/1(Kp_CoM) -> [Kp_CoM], Mux/1
  Gain Scheduling Function/2(Kd_CoM) -> [Kd_CoM], Mux/2
  Gain Scheduling Function/3(Kp_LFoot) -> [Kp_LFoot], Mux/3
  Gain Scheduling Function/4(Kd_LFoot) -> [Kd_LFoot], Mux/4
  Gain Scheduling Function/5(Kp_RFoot) -> [Kp_RFoot], Mux/5
  Gain Scheduling Function/6(Kd_RFoot) -> [Kd_RFoot], Mux/6
  Gain Scheduling Function/7(Kp_rot_task) -> [Kp_rot_task], Mux/7
  Gain Scheduling Function/8(Kd_rot_task) -> [Kd_rot_task], Mux/8
  Mux/1 -> Minimum Jerk Trajectory Generator5/1
  Gain Scheduling Function/9(impedances) -> [impedances], Mux/9
  Gain Scheduling Function/10(dampings) -> [dampings], Mux/10
  Gain Scheduling Function/11(smoothingTimeGains) -> Minimum Jerk Trajectory Generator5/2
  Minimum Jerk Trajectory Generator5/1 -> Demux/1
  Demux/1 -> Reshape/1
  Demux/2 -> Reshape1/1
  Demux/3 -> Reshape2/1
  Demux/4 -> Reshape3/1
  Reshape/1 -> Kp_Kd_CoM/1
  Reshape1/1 -> Kp_Kd_LFoot/1
  Reshape2/1 -> Kp_Kd_RFoot/1
  Reshape3/1 -> Kp_Kd_rot_task/1
  Demux/5 -> impedances/1
  Demux/6 -> dampings/1

== system torqueWalking/Robot State and References/Smooth References  ==
  state : Inport
  references_CoM : Inport  Port=2
  references_LFoot : Inport  Port=3
  references_RFoot : Inport  Port=4
  references_rot_task : Inport  Port=5
  references_s : Inport  Port=6
  Choose Smoothed or Direct References : Subsystem
  Selector1 : Selector  NumberOfDimensions=2  InputPortWidth=3  IndexOptions=Index vector (dialog),Index vector (dialog)  Indices=[1:3],1  OutputSizes=1,1
  Selector2 : Selector  NumberOfDimensions=2  InputPortWidth=3  IndexOptions=Index vector (dialog),Index vector (dialog)  Indices=[1:3],1  OutputSizes=1,1
  Selector4 : Selector  NumberOfDimensions=2  InputPortWidth=3  IndexOptions=Index vector (dialog),Index vector (dialog)  Indices=[1:3],[1:3]  OutputSizes=1,1
  Selector6 : Selector  NumberOfDimensions=2  InputPortWidth=3  IndexOptions=Index vector (dialog),Index vector (dialog)  Indices=[1:3],1  OutputSizes=1,1
  Selector7 : Selector  NumberOfDimensions=2  InputPortWidth=ROBOT_DOF  IndexOptions=Index vector (dialog),Index vector (dialog)  Indices=[1:ROBOT_DOF],1  OutputSizes=1,1
  Selector8 : Selector  NumberOfDimensions=2  InputPortWidth=3  IndexOptions=Index vector (dialog),Index vector (dialog)  Indices=[4:6],[1:3]  OutputSizes=1,1
  Selector9 : Selector  NumberOfDimensions=2  InputPortWidth=3  IndexOptions=Index vector (dialog),Index vector (dialog)  Indices=[4:6],[1:3]  OutputSizes=1,1
  Smooth Reference Orientations : Subsystem
  Smooth Reference Positions : Subsystem
  pos_vel_acc_CoM_des : Outport
  pose_vel_acc_LFoot_des : Outport  Port=2
  pose_vel_acc_RFoot_des : Outport  Port=3
  orient_vel_acc_rot_task_des : Outport  Port=4
  s_sDot_sDDot_ref : Outport  Port=5
  wires:
  references_CoM/1 -> Choose Smoothed or Direct References/5(references_CoM), Selector1/1
  Selector1/1 -> Smooth Reference Positions/1(pos_CoM_des)
  references_LFoot/1 -> Choose Smoothed or Direct References/6(references_LFoot), Selector9/1, Selector2/1
  Selector2/1 -> Smooth Reference Positions/2(pos_LFoot_des)
  references_RFoot/1 -> Selector8/1, Choose Smoothed or Direct References/7(references_RFoot), Selector6/1
  Selector6/1 -> Smooth Reference Positions/3(pos_RFoot_des)
  references_s/1 -> Choose Smoothed or Direct References/8(references_s), Selector7/1
  Selector7/1 -> Smooth Reference Positions/4(s_des)
  references_rot_task/1 -> Choose Smoothed or Direct References/9(references_rot_task), Selector4/1
  Selector4/1 -> Smooth Reference Orientations/3(w_R_Rot_task_des)
  Selector8/1 -> Smooth Reference Orientations/2(w_R_RFoot_des)
  Selector9/1 -> Smooth Reference Orientations/1(w_R_LFoot_des)
  Smooth Reference Positions/1(smooth_references_CoM) -> Choose Smoothed or Direct References/1(smooth_references_CoM)
  Smooth Reference Orientations/3(smooth_orient_vel_acc_Rot_task) -> Choose Smoothed or Direct References/12(smooth_references_rot_task)
  Smooth Reference Orientations/2(smooth_orient_vel_acc_RFoot) -> Choose Smoothed or Direct References/11(smooth_orient_vel_acc_RFoot)
  Smooth Reference Orientations/1(smooth_orient_vel_acc_LFoot) -> Choose Smoothed or Direct References/10(smooth_orient_vel_acc_LFoot)
  Choose Smoothed or Direct References/1(pos_vel_acc_CoM_des) -> pos_vel_acc_CoM_des/1
  Choose Smoothed or Direct References/2(pose_vel_acc_LFoot_des) -> pose_vel_acc_LFoot_des/1
  Choose Smoothed or Direct References/5(s_sDot_sDDot_ref) -> s_sDot_sDDot_ref/1
  Choose Smoothed or Direct References/4(orient_vel_acc_rot_task_des) -> orient_vel_acc_rot_task_des/1
  Choose Smoothed or Direct References/3(pose_vel_acc_RFoot_des) -> pose_vel_acc_RFoot_des/1
  state/1 -> Smooth Reference Positions/5(state), Smooth Reference Orientations/4(state)
  Smooth Reference Positions/2(smooth_pos_vel_acc_LFoot) -> Choose Smoothed or Direct References/2(smooth_pos_vel_acc_LFoot)
  Smooth Reference Positions/3(smooth_pos_vel_acc_RFoot) -> Choose Smoothed or Direct References/3(smooth_pos_vel_acc_RFoot)
  Smooth Reference Positions/4(smooth_references_s) -> Choose Smoothed or Direct References/4(smooth_references_s)

== system torqueWalking/Robot State and References/State Machines ==
  Base to Fixed Link Transform : Subsystem
  Compute State Velocity : Subsystem
  Constant6 : Constant  Value=eye(4)
  Get Estimate : WBToolboxLibrary/wholeBodyStates/Get Estimate  estimateType=Joints Position  robotName=WBT_robotName  localName=WBT_modelName  wbiFile=WBT_wbiFilename  wbiList=WBT_wbiList
      settings: SourceProductName=Whole Body Toolbox
  IMU measurements : WBToolboxLibrary/Utilities/Yarp Read  portName=Ports.IMU  signalSize=12  blocking=off  timestamp=off  autoconnect=on  errorOnConnection=off
      settings: SourceProductName=Whole Body Toolbox
  LFoot_is_fixed (walking) : WBToolboxLibrary/Utilities/Yarp Read  portName=PORTS.LFOOT_IS_FIXED  signalSize=1  blocking=off  timestamp=off  autoconnect=on  errorOnConnection=off
      settings: SourceProductName=Whole Body Toolbox
  Select the Current State and References : Subsystem
  Selector1 : Selector  NumberOfDimensions=2  InputPortWidth=ROBOT_DOF  IndexOptions=Index vector (dialog),Index vector (dialog)  Indices=[1:ROBOT_DOF],1  OutputSizes=1,1
  qt_fixed_LFoot (walking) : WBToolboxLibrary/Utilities/Yarp Read  portName=PORTS.LFOOT_DES  signalSize=7  blocking=off  timestamp=off  autoconnect=on  errorOnConnection=off
      settings: SourceProductName=Whole Body Toolbox
  "qt_fixed_RFoot (walking) " : WBToolboxLibrary/Utilities/Yarp Read  portName=PORTS.RFOOT_DES  signalSize=7  blocking=off  timestamp=off  autoconnect=on  errorOnConnection=off
      settings: SourceProductName=Whole Body Toolbox
  s : Outport
  w_H_b : Outport  Port=2
  nu : Outport  Port=3
  feetInContact : Outport  Port=4
  state : Outport  Port=5
  references_CoM : Outport  Port=6
  references_LFoot : Outport  Port=7
  references_RFoot : Outport  Port=8
  references_rot_task : Outport  Port=9
  references_s : Outport  Port=10
  tag scope: feetInContact=global, nu=global, s=global, s_des=global, state=global, w_H_b=global
  wires:
  Get Estimate/1 -> Base to Fixed Link Transform/1(s), Select the Current State and References/1(s), Compute State Velocity/1(s), s/1, [s]
  Constant6/1 -> Base to Fixed Link Transform/2(w_H_base_fixed)
  IMU measurements/1 -> Base to Fixed Link Transform/3(IMU port)
  qt_fixed_LFoot (walking)/1 -> Base to Fixed Link Transform/4(qt_fixed_LFoot (walking))
  LFoot_is_fixed (walking)/1 -> Base to Fixed Link Transform/5(LFoot_is_active (walking))
  "qt_fixed_RFoot (walking) "/1 -> Base to Fixed Link Transform/6(qt_fixed_RFoot (walking))
  Base to Fixed Link Transform/1(w_walking_H_LFoot) -> Select the Current State and References/2(w_walking_H_LFoot)
  Base to Fixed Link Transform/2(w_walking_H_RFoot) -> Select the Current State and References/3(w_walking_H_RFoot)
  Base to Fixed Link Transform/3(w_walking_H_b) -> Select the Current State and References/4(w_walking_H_b)
  Base to Fixed Link Transform/4(fixed_link_H_b) -> Select the Current State and References/5(fixed_link_H_b)
  Select the Current State and References/1(w_H_b) -> Compute State Velocity/2(w_H_b), w_H_b/1, [w_H_b]
  Select the Current State and References/2(feetInContact) -> Compute State Velocity/3("feetInContact "), feetInContact/1, [feetInContact]
  Compute State Velocity/1(nu) -> [nu], nu/1
  Select the Current State and References/3(state) -> [state], state/1
  Select the Current State and References/8(references_s) -> references_s/1, Selector1/1
  Select the Current State and References/4(references_CoM) -> references_CoM/1
  Select the Current State and References/7(references_rot_task) -> references_rot_task/1
  Select the Current State and References/6(references_RFoot) -> references_RFoot/1
  Select the Current State and References/5(references_LFoot) -> references_LFoot/1
  Selector1/1 -> [s_des]
  Base to Fixed Link Transform/5(LFoot_H_b) -> Select the Current State and References/6(LFoot_H_b)
  Base to Fixed Link Transform/6(RFoot_H_b) -> Select the Current State and References/7(RFoot_H_b)

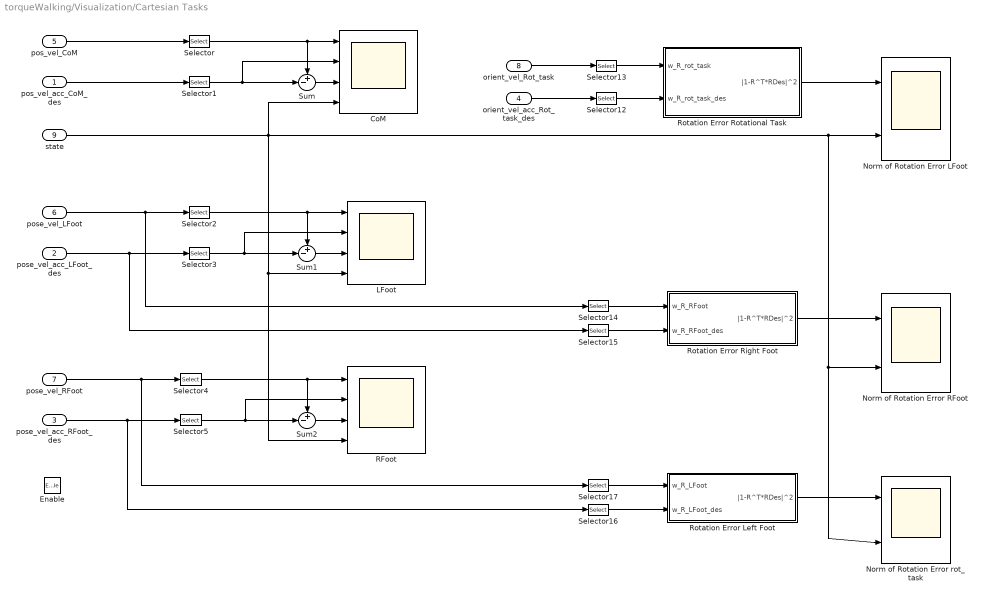
== system torqueWalking/Visualization/Cartesian Tasks ==
  pos_vel_acc_CoM_des : Inport
  pose_vel_acc_LFoot_des : Inport  Port=2
  pose_vel_acc_RFoot_des : Inport  Port=3
  orient_vel_acc_Rot_task_des : Inport  Port=4
  pos_vel_CoM : Inport  Port=5
  pose_vel_LFoot : Inport  Port=6
  pose_vel_RFoot : Inport  Port=7
  orient_vel_Rot_task : Inport  Port=8
  state : Inport  Port=9
  Enable : EnablePort
  CoM : Scope  NumInputPorts=4
  LFoot : Scope  NumInputPorts=4
  Norm of Rotation Error LFoot : Scope  NumInputPorts=2
  Norm of Rotation Error RFoot : Scope  NumInputPorts=2
  Norm of Rotation Error rot_task : Scope  NumInputPorts=2
  RFoot : Scope  NumInputPorts=4
  Rotation Error Left Foot : Subsystem
  Rotation Error Right Foot : Subsystem
  Rotation Error Rotational Task : Subsystem
  Selector{,1..5} (6 alike) : Selector  NumberOfDimensions=2  InputPortWidth=3  IndexOptions=Index vector (dialog),Index vector (dialog)  Indices=[1:3],1  OutputSizes=1,1
  Selector12 : Selector  NumberOfDimensions=2  InputPortWidth=3  IndexOptions=Index vector (dialog),Index vector (dialog)  Indices=[1:3],[1:3]  OutputSizes=1,1
  Selector13 : Selector  NumberOfDimensions=2  InputPortWidth=3  IndexOptions=Index vector (dialog),Index vector (dialog)  Indices=[1:3],[1:3]  OutputSizes=1,1
  Selector{14..17} (4 alike) : Selector  NumberOfDimensions=2  InputPortWidth=3  IndexOptions=Index vector (dialog),Index vector (dialog)  Indices=[4:6],[1:3]  OutputSizes=1,1
  Sum : Sum  Inputs=+-|
  Sum1 : Sum  Inputs=+-|
  Sum2 : Sum  Inputs=+-|
  wires:
  Selector1/1 -> CoM/2, Sum/2
  pos_vel_CoM/1 -> Selector/1
  pos_vel_acc_CoM_des/1 -> Selector1/1
  Selector2/1 -> Sum1/1, LFoot/1
  Selector3/1 -> Sum1/2, LFoot/2
  Selector4/1 -> Sum2/1, RFoot/1
  Selector5/1 -> RFoot/2, Sum2/2
  pose_vel_RFoot/1 -> Selector4/1, Selector17/1
  state/1 -> Norm of Rotation Error rot_task/2, Norm of Rotation Error RFoot/2, Norm of Rotation Error LFoot/2, CoM/4, RFoot/4, LFoot/4
  pose_vel_acc_RFoot_des/1 -> Selector5/1, Selector16/1
  pose_vel_LFoot/1 -> Selector2/1, Selector14/1
  Selector12/1 -> Rotation Error Rotational Task/2(w_R_rot_task_des)
  pose_vel_acc_LFoot_des/1 -> Selector15/1, Selector3/1
  orient_vel_acc_Rot_task_des/1 -> Selector12/1
  orient_vel_Rot_task/1 -> Selector13/1
  Selector/1 -> Sum/1, CoM/1
  Sum/1 -> CoM/3
  Sum1/1 -> LFoot/3
  Sum2/1 -> RFoot/3
  Rotation Error Rotational Task/1(|1-R^T*RDes|^2) -> Norm of Rotation Error LFoot/1
  Selector13/1 -> Rotation Error Rotational Task/1(w_R_rot_task)
  Rotation Error Right Foot/1(|1-R^T*RDes|^2) -> Norm of Rotation Error RFoot/1
  Selector14/1 -> Rotation Error Right Foot/1(w_R_RFoot)
  Selector15/1 -> Rotation Error Right Foot/2(w_R_RFoot_des)
  Rotation Error Left Foot/1(|1-R^T*RDes|^2) -> Norm of Rotation Error rot_task/1
  Selector16/1 -> Rotation Error Left Foot/2(w_R_LFoot_des)
  Selector17/1 -> Rotation Error Left Foot/1(w_R_LFoot)
